simulink model "Complete_HPP_Model_PEM_WIndTurbine"  (R2022a)
settings: Solver=ode4  StartTime=0.0  StopTime=5  FixedStep=1e-6  MaxStep=50e-7  RelTol=1e-3
undefined symbols (not defined in the file or in its folder): DiscIntNeverNeededParam, Ts_Control
libraries: spsMeanLib x9, spsSeriesRLCBranchLib x8, spsIGBTDiodeLib x7, spsVoltageMeasurementLib x6, spsThreePhaseVIMeasurementLib x4, spsDiodeLib x4, spsCurrentMeasurementLib x4, spsMosfetLib x3, spsThreePhaseSeriesRLCBranchLib x2, spsGroundLib x2, spsSawtoothGeneratorLib x2, spsWindTurbineLib x1
(part 2 of 2)

== system Complete_HPP_Model_PEM_WIndTurbine/Electrolyzer Complete Mathematical Model with Storage tank /Dynamic activation losses ==
  I : Inport
  Vcon : Inport  Port=2
  V_activation_steady : Inport  Port=3
  . : Sum  Inputs=|++
  .1 : Sum  Inputs=|+-
  Constant : Constant
  Discrete-Time Integrator : DiscreteIntegrator  SampleTime=1e-6  ICPrevOutput=DiscIntNeverNeededParam  ICPrevScaledInput=DiscIntNeverNeededParam
  Divide1 : Product  Inputs=*/
  Divide2 : Product  Inputs=/*
  Divide3 : Product  Inputs=/*
  Product : Product
  vact : Outport
  wires:
  ./1 -> Divide2/2
  Discrete-Time Integrator/1 -> Divide3/2, vact/1
  I/1 -> Divide1/1, Divide2/1
  Divide1/1 -> .1/1
  .1/1 -> Discrete-Time Integrator/1
  Constant/1 -> Product/1, Divide1/2
  V_activation_steady/1 -> ./2
  Vcon/1 -> ./1
  Divide2/1 -> Product/2
  Divide3/1 -> .1/2
  Product/1 -> Divide3/1

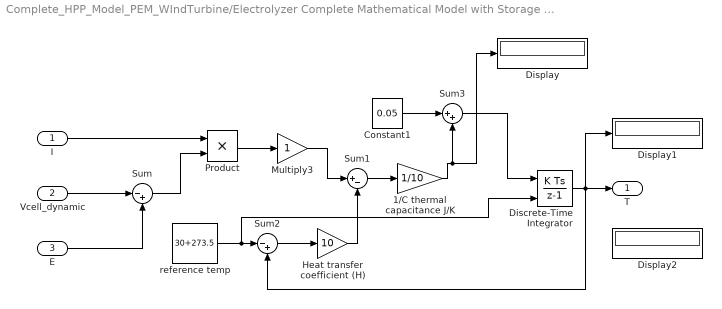
== system Complete_HPP_Model_PEM_WIndTurbine/Electrolyzer Complete Mathematical Model with Storage tank /Dynamic temperature model ==
  I : Inport
  Vcell_dynamic : Inport  Port=2
  E : Inport  Port=3
  1/C thermal capacitance J/K : Gain  Gain=1/10
  Constant1 : Constant  Value=0.05
  Discrete-Time Integrator : DiscreteIntegrator  InitialConditionSource=external  InitialCondition=0.001  SampleTime=1e-6  ICPrevOutput=DiscIntNeverNeededParam  ICPrevScaledInput=DiscIntNeverNeededParam
  Display : Display
  Display1 : Display
  Display2 : Display
  Heat transfer coefficient (H) : Gain  Gain=10
  Multiply3 : Gain
  Product : Product
  Sum : Sum  Inputs=|-+
  Sum1 : Sum  Inputs=|+-
  Sum2 : Sum  Inputs=|-+
  Sum3 : Sum  Inputs=|++
  reference temp : Constant  Value=30+273.5
  T : Outport
  wires:
  Multiply3/1 -> Sum1/1
  Product/1 -> Multiply3/1
  Discrete-Time Integrator/1 -> Sum2/2, Display1/1, T/1
  Sum2/1 -> Heat transfer coefficient (H)/1
  I/1 -> Product/1
  Vcell_dynamic/1 -> Sum/1
  Sum/1 -> Product/2
  E/1 -> Sum/2
  Sum1/1 -> 1/C thermal capacitance J/K/1
  Heat transfer coefficient (H)/1 -> Sum1/2
  reference temp/1 -> Discrete-Time Integrator/2, Sum2/1
  1/C thermal capacitance J/K/1 -> Display/1, Sum3/2
  Constant1/1 -> Sum3/1
  Sum3/1 -> Discrete-Time Integrator/1

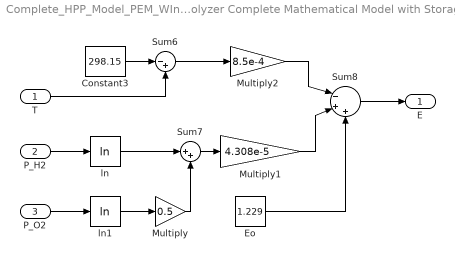
== system Complete_HPP_Model_PEM_WIndTurbine/Electrolyzer Complete Mathematical Model with Storage tank /Ernest cell Voltage ==
  T : Inport
  P_H2 : Inport  Port=2
  P_O2 : Inport  Port=3
  Constant3 : Constant  Value=298.15
  Eo : Constant  Value=1.229
  Multiply : Gain  Gain=0.5
  Multiply1 : Gain  Gain=4.308e-5
  Multiply2 : Gain  Gain=8.5e-4
  Sum6 : Sum  Inputs=|-+
  Sum7 : Sum  Inputs=|++
  Sum8 : Sum  Inputs=|-++
  ln : Math  Operator=log
  ln1 : Math  Operator=log
  E : Outport
  wires:
  Constant3/1 -> Sum6/1
  Sum6/1 -> Multiply2/1
  ln1/1 -> Multiply/1
  Eo/1 -> Sum8/3
  Multiply1/1 -> Sum8/2
  Sum8/1 -> E/1
  Sum7/1 -> Multiply1/1
  Multiply/1 -> Sum7/2
  P_H2/1 -> ln/1
  T/1 -> Sum6/2
  ln/1 -> Sum7/1
  P_O2/1 -> ln1/1
  Multiply2/1 -> Sum8/1

== system Complete_HPP_Model_PEM_WIndTurbine/Electrolyzer Complete Mathematical Model with Storage tank /Ohmic losses ==
  I : Inport
  T : Inport  Port=2
  . : Sum  Inputs=|+-+
  Constant3 : Constant  Value=1.605e-2
  Multiply : Gain  Gain=8e-5
  Multiply1 : Gain  Gain=3.5e-5
  Multiply2 : Gain  Gain=-1
  Product : Product
  nohm : Outport
  wires:
  Product/1 -> nohm/1
  Multiply1/1 -> ./2
  I/1 -> Multiply2/1, Multiply/1
  Multiply/1 -> ./1
  Multiply2/1 -> Product/1
  ./1 -> Product/2
  Constant3/1 -> ./3
  T/1 -> Multiply1/1

== system Complete_HPP_Model_PEM_WIndTurbine/Electrolyzer Complete Mathematical Model with Storage tank /Oxygen concetration ==
  T : Inport
  P_O2 : Inport  Port=2
  Constant3 : Constant  Value=-498
  Constant4 : Constant  Value=5.08e6
  Divide1 : Product  Inputs=/*
  Divide2 : Product  Inputs=*/
  Exp : Math
  Product : Product
  Con_O2 : Outport
  wires:
  Exp/1 -> Product/1
  P_O2/1 -> Divide1/2
  Constant3/1 -> Divide2/1
  Divide1/1 -> Con_O2/1
  T/1 -> Divide2/2
  Constant4/1 -> Product/2
  Product/1 -> Divide1/1
  Divide2/1 -> Exp/1

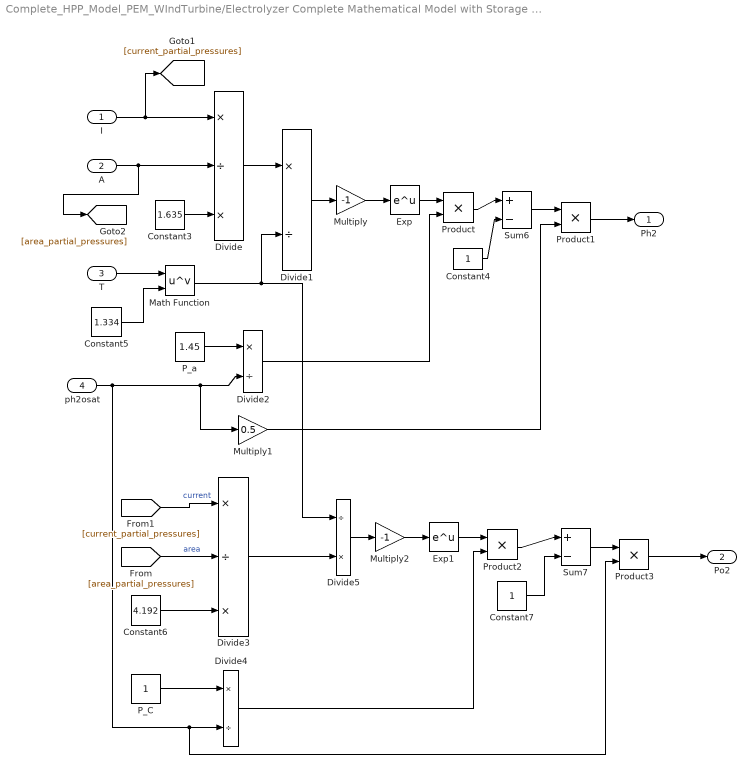
== system Complete_HPP_Model_PEM_WIndTurbine/Electrolyzer Complete Mathematical Model with Storage tank /Partial pressures ==
  I : Inport
  A : Inport  Port=2
  T : Inport  Port=3
  ph2osat : Inport  Port=4
  Constant3 : Constant  Value=1.635
  Constant4 : Constant
  Constant5 : Constant  Value=1.334
  Constant6 : Constant  Value=4.192
  Constant7 : Constant
  Divide : Product  Inputs=*/*
  Divide1 : Product  Inputs=*/
  Divide2 : Product  Inputs=*/
  Divide3 : Product  Inputs=*/*
  Divide4 : Product  Inputs=*/
  Divide5 : Product  Inputs=/*
  Exp : Math
  Exp1 : Math
  Math Function : Math  Operator=pow
  Multiply : Gain  Gain=-1
  Multiply1 : Gain  Gain=0.5
  Multiply2 : Gain  Gain=-1
  P_C : Constant
  P_a : Constant  Value=1.45
  Product{,1..3} (4 alike) : Product
  Sum6 : Sum  Inputs=|+-
  Sum7 : Sum  Inputs=|+-
  Ph2 : Outport
  Po2 : Outport  Port=2
  wires:
  Constant5/1 -> Math Function/2
  Constant7/1 -> Sum7/2
  Constant6/1 -> Divide3/3
  Constant4/1 -> Sum6/2
  ph2osat/1 -> Multiply1/1, Divide2/2, Product3/2, Divide4/2
  Divide5/1 -> Multiply2/1
  A/1 -> [area_partial_pressures], Divide/2
  T/1 -> Math Function/1
  Product2/1 -> Sum7/1
  Divide3/1 -> Divide5/2
  Product1/1 -> Ph2/1
  Exp/1 -> Product/1
  Constant3/1 -> Divide/3
  I/1 -> [current_partial_pressures], Divide/1
  Multiply/1 -> Exp/1
  P_C/1 -> Divide4/1
  Math Function/1 -> Divide5/1, Divide1/2
  Sum7/1 -> Product3/1
  [current_partial_pressures] -> Divide3/1  "current"
  Multiply1/1 -> Product1/2
  Multiply2/1 -> Exp1/1
  Exp1/1 -> Product2/1
  Divide1/1 -> Multiply/1
  Divide/1 -> Divide1/1
  Sum6/1 -> Product1/1
  Product/1 -> Sum6/1
  Divide4/1 -> Product2/2
  P_a/1 -> Divide2/1
  [area_partial_pressures] -> Divide3/2  "area"
  Product3/1 -> Po2/1
  Divide2/1 -> Product/2

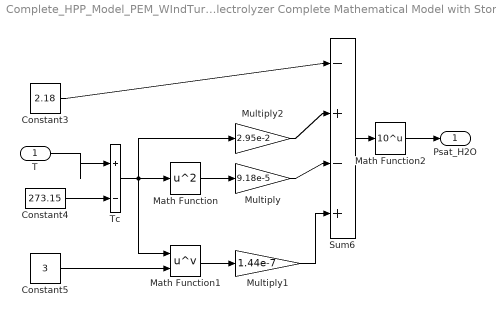
== system Complete_HPP_Model_PEM_WIndTurbine/Electrolyzer Complete Mathematical Model with Storage tank /Saturation pressure H2O ==
  T : Inport
  Constant3 : Constant  Value=2.18
  Constant4 : Constant  Value=273.15
  Constant5 : Constant  Value=3
  Math Function : Math  Operator=square
  Math Function1 : Math  Operator=pow
  Math Function2 : Math  Operator=10^u
  Multiply : Gain  Gain=9.18e-5
  Multiply1 : Gain  Gain=1.44e-7
  Multiply2 : Gain  Gain=2.95e-2
  Sum6 : Sum  Inputs=|-+-+
  Tc : Sum  Inputs=|+-
  Psat_H2O : Outport
  wires:
  Multiply1/1 -> Sum6/4
  Constant3/1 -> Sum6/1
  Math Function2/1 -> Psat_H2O/1
  Math Function/1 -> Multiply/1
  Constant5/1 -> Math Function1/2
  Tc/1 -> Multiply2/1, Math Function/1, Math Function1/1
  Sum6/1 -> Math Function2/1
  Multiply/1 -> Sum6/3
  T/1 -> Tc/1
  Math Function1/1 -> Multiply1/1
  Multiply2/1 -> Sum6/2
  Constant4/1 -> Tc/2

== system Complete_HPP_Model_PEM_WIndTurbine/Electrolyzer Complete Mathematical Model with Storage tank /Steady state activation losses ==
  T : Inport
  I : Inport  Port=2
  Con_O2 : Inport  Port=3
  Constant3 : Constant  Value=0.9514
  Exp : Math  Operator=log
  Exp1 : Math  Operator=log
  Multiply : Gain  Gain=1.87e-4
  Multiply1 : Gain  Gain=7.4e-5
  Multiply2 : Gain  Gain=3.12e-3
  Product : Product
  Product1 : Product
  Sum6 : Sum  Inputs=|-+-+
  n_act : Outport
  wires:
  T/1 -> Product1/2, Product/2, Multiply2/1
  Product1/1 -> Sum6/4
  Constant3/1 -> Sum6/1
  Con_O2/1 -> Exp1/1
  Exp1/1 -> Multiply1/1
  I/1 -> Exp/1
  Exp/1 -> Multiply/1
  Multiply1/1 -> Product1/1
  Multiply/1 -> Product/1
  Multiply2/1 -> Sum6/2
  Sum6/1 -> n_act/1
  Product/1 -> Sum6/3

== system Complete_HPP_Model_PEM_WIndTurbine/PWM generator for Electrolyser/PWM signal creator3 ==
  "Vcontrol input " : Inport
  1V peak to peak : spsSawtoothGeneratorLib/Sawtooth Generator  Freq=Fs  Phase=0  Ts=Ts
  Add dc offset : Constant
  Divide1 : Product  Inputs=*/
  Relational Operator : RelationalOperator  Operator=<=  OutDataTypeStr=boolean  RndMeth=Simplest  InputSameDT=off
  Scope11 : Scope  NumInputPorts=3
  Sum1 : Sum  Inputs=|++
  make 0-1V : Constant  Value=2
  PWM signal : Outport
  wires:
  Sum1/1 -> Divide1/1
  Divide1/1 -> Scope11/1, Relational Operator/1  "sawtooth"
  Relational Operator/1 -> PWM signal/1, Scope11/3  "pwm"
  1V peak to peak/1 -> Sum1/1
  "Vcontrol input "/1 -> Relational Operator/2, Scope11/2  "vcontrol"
  make 0-1V/1 -> Divide1/2
  Add dc offset/1 -> Sum1/2

== matlab function Complete_HPP_Model_PEM_WIndTurbine/12.3 kW wind turbine complete model/Control of operation of wind turbine/Cutt off on wind speed ==
  data: u input; y output
function y = fcn(u)
x=0;  
  if u>17 %%cut off wind speed
     x=1;
  end
  if u<5 %% shut down
     x=1;
  end
y = x;

== matlab function Complete_HPP_Model_PEM_WIndTurbine/MPPT Control perturb and observe   ==
  settings: updateMethod=DISCRETE  sampleTime=Ts_Control
  data: Param input; Enabled input; V input =V; I input; D output
function D  = PandO(Param, Enabled, V, I)

Dinit = Param(1);  %Initial value for D output
Dmax = Param(2);   %Maximum value for D
Dmin = Param(3);   %Minimum value for D
deltaD = Param(4); %Increment value used to increase/decrease the duty cycle D
% ( increasing D = decreasing Vref )
%  

persistent Vold Pold Dold;

dataType = 'double';

if isempty(Vold)
    Vold=0;
    Pold=0;
    Dold=Dinit;
end
P= V*I;
dV= V - Vold;
dP= P - Pold;

if dP ~= 0 & Enabled ~=0
    if dP < 0
        if dV < 0
            D = Dold - deltaD;
        else
            D = Dold + deltaD;
        end
    else
        if dV < 0
            D = Dold + deltaD;
        else
            D = Dold - deltaD;
        end    
    end
else D=Dold;
end

if D >= Dmax | D<= Dmin
    D=Dold;
end

Dold=D;
Vold=V;
Pold=P;
